simulink model "MCC_retour_etat"  (R2024a)
settings: Solver=ode45  StartTime=0.0  StopTime=Tfinal  RelTol=1e-3
undefined symbols (not defined in the file): A, B_sim, C, D_sim, K, Nr, Tmec, x0
settings Model: Creator=DELL  LastModifiedBy=DELL

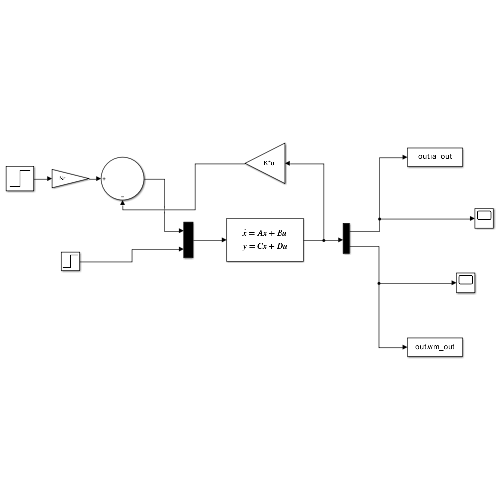
[thumbnail: Simulink's stored preview of the top-level diagram]
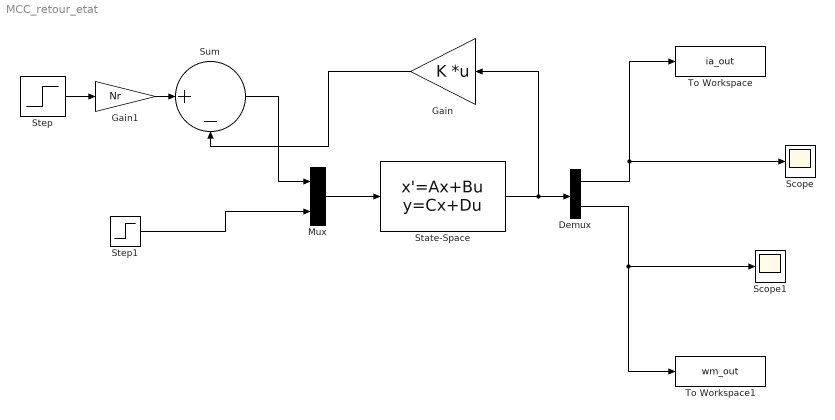
== system MCC_retour_etat ==
  Demux : Demux  Outputs=2
  Gain : Gain  Gain=K  Multiplication=Matrix(K*u)
  Gain1 : Gain  Gain=Nr
  Mux : Mux  Inputs=2
  Scope : Scope
  Scope1 : Scope
  State-Space : StateSpace  A=A  B=B_sim  C=C  D=D_sim  InitialCondition=x0
  Step : Step  Time=0.1  After=190  SampleTime=0
  Step1 : Step  Time=0.5  After=Tmec  SampleTime=0
  Sum : Sum  Inputs=|+-
  To Workspace : ToWorkspace  VariableName=ia_out  SaveFormat=Timeseries  SampleTime=-1
  To Workspace1 : ToWorkspace  VariableName=wm_out  SaveFormat=Timeseries  SampleTime=-1
  wires:
  Mux/1 -> State-Space/1
  Step1/1 -> Mux/2
  Demux/1 -> Scope/1, To Workspace/1
  Demux/2 -> To Workspace1/1, Scope1/1
  Sum/1 -> Mux/1
  Gain/1 -> Sum/2
  State-Space/1 -> Gain/1, Demux/1
  Step/1 -> Gain1/1
  Gain1/1 -> Sum/1
